simulink model "schematico_per_screen"  (R2020a)
settings: Solver=VariableStepAuto  StartTime=0.0  StopTime=10.0  RelTol=1e-3
settings Model: Creator=augus  LastModifiedBy=augus

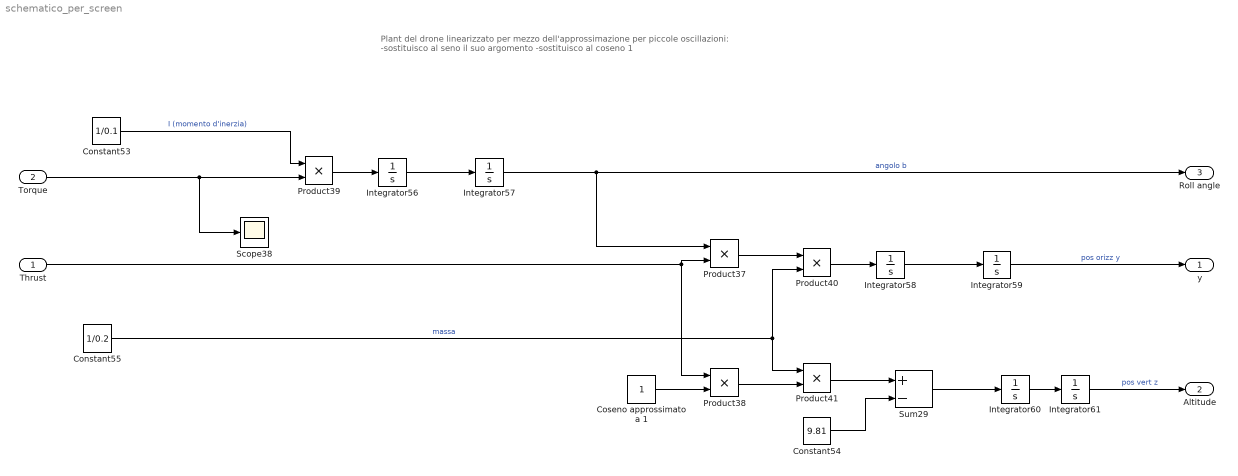
== system schematico_per_screen ==
  note: Plant del drone linearizzato per mezzo dell'approssimazione per piccole oscillazioni:
      | -sostituisco al seno il suo argomento
      | -sostituisco al coseno 1
  Thrust : Inport  Tag=torque  Description=torque
  Torque : Inport  Tag=thrust  Description=thrust  Port=2
  Constant53 : Constant  Value=1/0.1
  Constant54 : Constant  Value=9.81
  Constant55 : Constant  Value=1/0.2
  Coseno approssimato a 1 : Constant
  Integrator{56..61} (6 alike) : Integrator
  Product{37..41} (5 alike) : Product
  Scope38 : Scope
  Sum29 : Sum  Inputs=+-
  y : Outport  Tag=y position  Description=y position
  Altitude : Outport  Tag=z position  Description=z position  Port=2
  Roll angle : Outport  Tag=roll angle  Description=roll angle  Port=3
  wires:
  Product39/1 -> Integrator56/1
  Integrator59/1 -> y/1  "pos orizz y"
  Product41/1 -> Sum29/1
  Constant53/1 -> Product39/1  "I (momento d'inerzia)"
  Coseno approssimato a 1/1 -> Product38/2
  Integrator61/1 -> Altitude/1  "pos vert z"
  Constant54/1 -> Sum29/2
  Thrust/1 -> Product38/1, Product37/2
  Product38/1 -> Product41/2
  Torque/1 -> Scope38/1, Product39/2
  Product37/1 -> Product40/1
  Sum29/1 -> Integrator60/1
  Integrator56/1 -> Integrator57/1
  Constant55/1 -> Product40/2, Product41/1  "massa"
  Integrator58/1 -> Integrator59/1
  Integrator60/1 -> Integrator61/1
  Integrator57/1 -> Product37/1, Roll angle/1  "angolo b"
  Product40/1 -> Integrator58/1
